simulink model "ex5model"  (R2022b)
settings: Solver=FixedStepAuto  StartTime=0.0  StopTime=10  FixedStep=0.001  RelTol=1e-3
values from neighbouring files (symbols this model uses):
  a21 = 1/(2*m)*x30^2*FemP1/FemP2^2*exp(-x10/FemP2)    [ex5.m]
  a23 = -1/(m)*x30*FemP1/FemP2*exp(-x10/FemP2)    [ex5.m]
  a31 = 1/f1*exp(x10/f2)*(ki*u10+ci-x30)    [ex5.m]
  a33 = -f2/f1*exp(x10/f2)    [ex5.m]
  b31 = ki*f2/f1*exp(x10/f2)    [ex5.m]
  g = 9.81    [ex5.m]
  Kx = -acker(A, B(:,1), -sKx)    [ex5.m]
  Lo = acker(A', C', -sLo)    [ex5.m]
  u0 = -(a31*x1+a33*x3)/b31    [ex5.m]
  x1 = .003    (= 0.003)    [ex5.m]
  x2 = 0    [ex5.m]
  x3 = -(a21*x1+g)/a23    [ex5.m]
  xd = d-bd    (= 0.0192)    [ex5.m]
settings Model: Creator=AgraWoodAdmin  LastModifiedBy=MPatr
settings DebuggingCC: UnconnectedInputMsg=warning  UnconnectedOutputMsg=warning  UnconnectedLineMsg=warning
settings ModelReferenceCC: EnableRefExpFcnMdlSchedulingChecks=on
settings RTWCC: DLArmComputeVersion=19.05

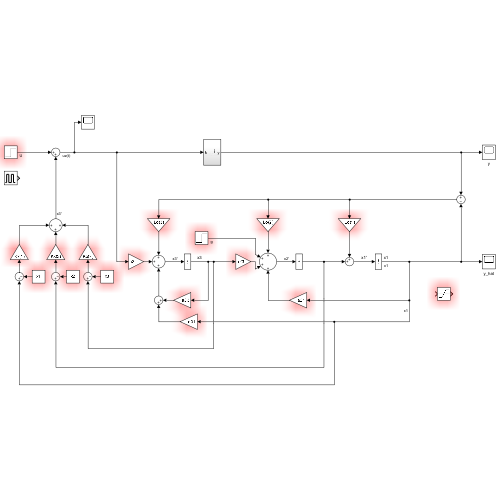
[thumbnail: Simulink's stored preview of the top-level diagram]
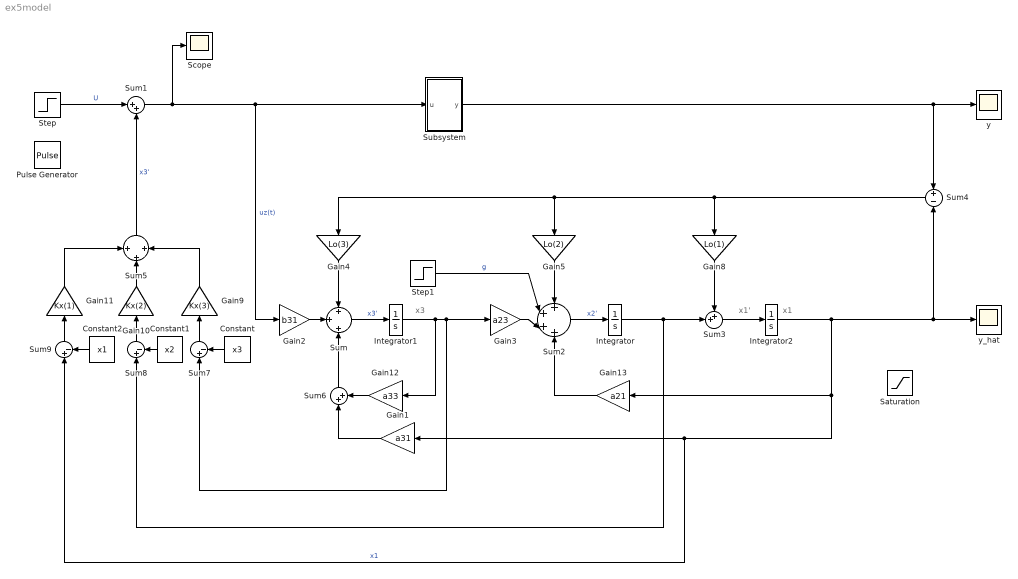
== system ex5model ==
  note: x3
  note: x1'
  note: x1
  Constant : Constant  Value=x3
  Constant1 : Constant  Value=x2
  Constant2 : Constant  Value=x1
  Gain1 : Gain  Gain=a31
  Gain10 : Gain  Gain=Kx(2)
  Gain11 : Gain  Gain=Kx(1)
  Gain12 : Gain  Gain=a33
  Gain13 : Gain  Gain=a21
  Gain2 : Gain  Gain=b31
  Gain3 : Gain  Gain=a23
  Gain4 : Gain  Gain=Lo(3)
  Gain5 : Gain  Gain=Lo(2)
  Gain8 : Gain  Gain=Lo(1)
  Gain9 : Gain  Gain=Kx(3)
  Integrator : Integrator  InitialCondition=40
  Integrator1 : Integrator  InitialCondition=20
  Integrator2 : Integrator  InitialCondition=40
  Pulse Generator : DiscretePulseGenerator  PulseType=Time based  Amplitude=0  Period=10
  Saturation : Saturate  UpperLimit=xd  LowerLimit=0
  Scope : Scope
  Step : Step  Time=0  After=u0  SampleTime=0
  Step1 : Step  Time=0  After=g  SampleTime=0
  Subsystem : Subsystem
  Sum : Sum  Inputs=+|+|+
  Sum1 : Sum  Inputs=|++
  Sum2 : Sum  Inputs=+|+|+|+
  Sum3 : Sum  Inputs=++|
  Sum4 : Sum  Inputs=+|-
  Sum5 : Sum  Inputs=+|+|+
  Sum6 : Sum  Inputs=|++
  Sum7 : Sum  Inputs=|+-
  Sum8 : Sum  Inputs=|+-
  Sum9 : Sum  Inputs=|+-
  y : Scope
  y_hat : Scope
  wires:
  Step/1 -> Sum1/1  "U"
  Gain4/1 -> Sum/1
  Sum4/1 -> Gain4/1, Gain5/1, Gain8/1
  Subsystem/1(y) -> y/1, Sum4/1
  Gain2/1 -> Sum/2
  Sum2/1 -> Integrator/1  "x2'"
  Gain1/1 -> Sum6/1
  Sum/1 -> Integrator1/1  "x3'"
  Gain3/1 -> Sum2/3
  Gain5/1 -> Sum2/1
  Sum1/1 -> Scope/1, Subsystem/1(u), Gain2/1  "uz(t)"
  Sum3/1 -> Integrator2/1
  Gain8/1 -> Sum3/1
  Sum5/1 -> Sum1/2  "x3'"
  Integrator1/1 -> Gain12/1, Gain3/1, Sum7/1
  Integrator/1 -> Sum3/2, Sum8/1
  Sum6/1 -> Sum/3
  Gain12/1 -> Sum6/2
  Gain13/1 -> Sum2/4
  Integrator2/1 -> y_hat/1, Sum4/2, Gain13/1, Sum9/1, Gain1/1  "x1"
  Step1/1 -> Sum2/2  "g"
  Constant/1 -> Sum7/2
  Sum7/1 -> Gain9/1
  Constant1/1 -> Sum8/2
  Sum8/1 -> Gain10/1
  Constant2/1 -> Sum9/2
  Sum9/1 -> Gain11/1
  Gain9/1 -> Sum5/3
  Gain10/1 -> Sum5/2
  Gain11/1 -> Sum5/1

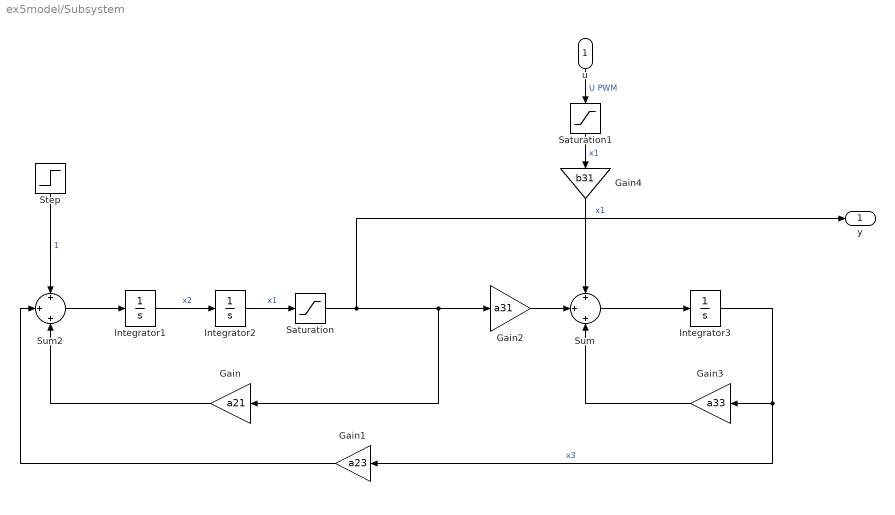
== system ex5model/Subsystem ==
  u : Inport
  Gain : Gain  Gain=a21
  Gain1 : Gain  Gain=a23
  Gain2 : Gain  Gain=a31
  Gain3 : Gain  Gain=a33
  Gain4 : Gain  Gain=b31
  Integrator1 : Integrator
  Integrator2 : Integrator
  Integrator3 : Integrator
  Saturation : Saturate  UpperLimit=xd  LowerLimit=0
  Saturation1 : Saturate  UpperLimit=1  LowerLimit=0
  Step : Step  Time=0  After=g  SampleTime=0
  Sum : Sum  Inputs=+|+|+
  Sum2 : Sum  Inputs=+|+|+
  y : Outport
  wires:
  Step/1 -> Sum2/1  "1"
  Integrator1/1 -> Integrator2/1  "x2"
  Gain1/1 -> Sum2/2
  u/1 -> Saturation1/1  "U PWM"
  Saturation/1 -> y/1, Gain2/1, Gain/1  "x1"
  Integrator3/1 -> Gain3/1, Gain1/1  "x3"
  Gain/1 -> Sum2/3
  Gain2/1 -> Sum/2
  Gain3/1 -> Sum/3
  Sum2/1 -> Integrator1/1
  Sum/1 -> Integrator3/1
  Integrator2/1 -> Saturation/1  "x1"
  Gain4/1 -> Sum/1
  Saturation1/1 -> Gain4/1  "x1"
